simulink model "Model_without_decision_and_sieve"  (R2022a)
settings: Solver=VariableStepAuto  StartTime=0.0  StopTime=1000000  RelTol=1e-3
undefined symbols (not defined in the file): Coefficient_value, Enable_X, Enable_Y, N, s1, s10, s11, s12, s13, s14, s15, s16, s17, s18, s19, s2, s20, s21, s22, s23, s24, s25, s26, s27, s28, s29, s3, s30, s4, s5, s6, s7, s8, s9
libraries: simulink x33
(part 1 of 5)
settings Model: Creator=jhd  LastModifiedBy=AISL
settings SolverCC: AlgebraicLoopSolver=TrustRegion
settings DebuggingCC: UnconnectedInputMsg=warning  UnconnectedOutputMsg=warning  UnconnectedLineMsg=warning  SFMachineParentedDataDiag=warning
settings RTWCC: DLArmComputeVersion=19.05

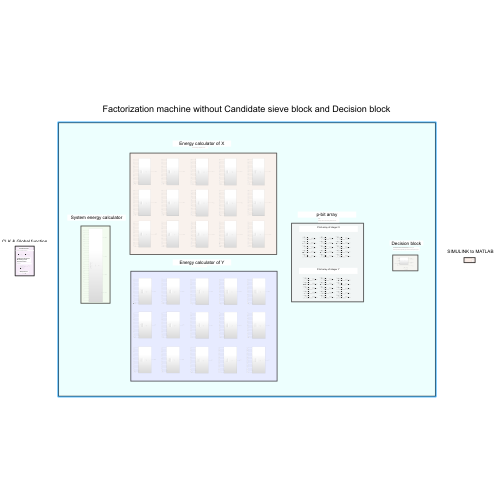
[thumbnail: Simulink's stored preview of the top-level diagram]
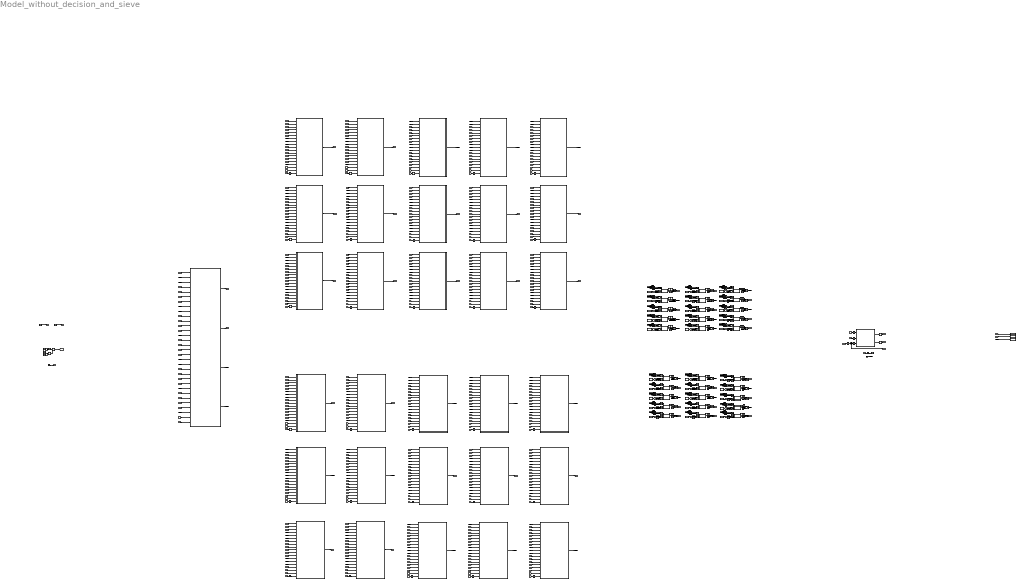
== system Model_without_decision_and_sieve ==
  note: Coefficient value and Bit-shifting of the energy function
  note: UPDATING CLK
  note: P-bit array of integer X
  note: P-bit array of integer Y
  note: CLK & Global function
  note: System energy calculator
  note: Energy calculator of X
  note: Energy calculator of Y
  note: SIMULINK to MATLAB
  note: Decision block
  note: Semiprime N
  note: p-bit array
  note: EN_X, EN_Y, which are signals for updating p-bits.
  note: Calculates the energy for updating the p-bits of X
  note: Calculates the energy for updating the p-bits of Y
  note: When the EN_X(EN_Y) signal rises, the p-bits are updated by the sigmoid function and RNG.
      |
      | Unnecessary number of p-bits for factorizing given N are fixed to zero.
  note: When both X and Y are the factors of semiprime number N, the system energy is 0.
      | Then, the Find signal becomes zero and the simulation stops.
      |
      | In the Enable_switch block, the EN_X and EN_Y signals are fixed to zero when the system energy is 0.
  note: A coefficient value E 0 and bit-shifting operation by the probabilistic annealing method.
  note: Factorization machine without Candidate sieve block and Decision block
  Clock : Clock
  Constant{1..4,6..7,9,11..18,21,29,33,39,57..58,60..61,63..64,66,68..70,72..73,75..76,78..79,81,83,85,87,95,99,101,103..104,106,111,113,117..119,121,123..124,150..151,153..155,195..196} (60 alike) : Constant  Value=0
  Constant10 : Constant  Value=Enable_X(13,1)
  Constant100 : Constant  Value=Enable_X(4,1)
  Constant102 : Constant  Value=Enable_X(3,1)
  Constant105 : Constant  Value=Enable_X(1,1)
  Constant112 : Constant  Value=Enable_X(5,1)
  Constant116 : Constant  Value=Enable_X(2,1)
  Constant120 : Constant  Value=Enable_Y(14,1)
  Constant122 : Constant  Value=Enable_Y(13,1)
  Constant131 : Constant  Value=2
  Constant149 : Constant  Value=Enable_Y(11,1)
  Constant152 : Constant  Value=Enable_Y(12,1)
  Constant194 : Constant  Value=Enable_Y(15,1)
  Constant20 : Constant  Value=Enable_X(11,1)
  Constant22 : Constant  Value=2
  Constant23 : Constant  Value=Coefficient_value
  Constant28 : Constant  Value=Enable_X(15,1)
  Constant32 : Constant  Value=Enable_X(12,1)
  Constant34 : Constant  Value=Enable_X(9,1)
  Constant36 : Constant  Value=Enable_X(8,1)
  Constant5 : Constant  Value=N
  Constant56 : Constant  Value=Enable_Y(4,1)
  Constant59 : Constant  Value=Enable_Y(3,1)
  Constant62 : Constant  Value=Enable_Y(1,1)
  Constant65 : Constant  Value=Enable_Y(5,1)
  Constant67 : Constant  Value=Enable_Y(2,1)
  Constant71 : Constant  Value=Enable_Y(9,1)
  Constant74 : Constant  Value=Enable_Y(8,1)
  Constant77 : Constant  Value=Enable_Y(6,1)
  Constant8 : Constant  Value=Enable_X(14,1)
  Constant80 : Constant  Value=Enable_Y(10,1)
  Constant82 : Constant  Value=Enable_Y(7,1)
  Constant86 : Constant  Value=Enable_X(6,1)
  Constant94 : Constant  Value=Enable_X(10,1)
  Constant98 : Constant  Value=Enable_X(7,1)
  Delay{1..13,17,27..32,34..42,49} (30 alike) : Delay  DelayLength=1
  Enable_Switch : Subsystem
  Logical Operator2 : Logic  Operator=NOT  Inputs=1  AllPortsSameDT=off  OutDataTypeStr=boolean
  Math Function1 : Math  Operator=pow
  Math Function2 : Math  Operator=pow
  Pbit_1 : Subsystem
  Pbit_10 : Subsystem
  Pbit_11 : Subsystem
  Pbit_12 : Subsystem
  Pbit_13 : Subsystem
  Pbit_14 : Subsystem
  Pbit_15 : Subsystem
  Pbit_2 : Subsystem
  Pbit_3 : Subsystem
  Pbit_4 : Subsystem
  Pbit_5 : Subsystem
  Pbit_6 : Subsystem
  Pbit_7 : Subsystem
  Pbit_8 : Subsystem
  Pbit_9 : Subsystem
  Pbit_Y_1 : Subsystem
  Pbit_Y_10 : Subsystem
  Pbit_Y_11 : Subsystem
  Pbit_Y_12 : Subsystem
  Pbit_Y_13 : Subsystem
  Pbit_Y_14 : Subsystem
  Pbit_Y_15 : Subsystem
  Pbit_Y_2 : Subsystem
  Pbit_Y_3 : Subsystem
  Pbit_Y_4 : Subsystem
  Pbit_Y_5 : Subsystem
  Pbit_Y_6 : Subsystem
  Pbit_Y_7 : Subsystem
  Pbit_Y_8 : Subsystem
  Pbit_Y_9 : Subsystem
  Product1 : Product
  Repeating Sequence Stair : simulink/Sources/Repeating Sequence Stair  OutValues=[0 1 2 3].'  tsamp=6  OutMin=[]  OutMax=[]  OutDataTypeStr=double  OutputDataTypeScalingMode=double  OutDataType=fixdt(0,8)  ConRadixGroup=Best Precision: Vector-wise  OutScaling=2^-12
  Repeating Sequence Stair1 : simulink/Sources/Repeating Sequence Stair  OutValues=[1 0 0 0 0 0].'  tsamp=1  OutMin=[]  OutMax=[]  OutDataTypeStr=double  OutputDataTypeScalingMode=double  OutDataType=fixdt(0,8)  ConRadixGroup=Best Precision: Vector-wise  OutScaling=2^-12
  Repeating Sequence Stair2 : simulink/Sources/Repeating Sequence Stair  OutValues=[0 0 0 1 0 0 ].'  tsamp=1  OutMin=[]  OutMax=[]  OutDataTypeStr=double  OutputDataTypeScalingMode=double  OutDataType=fixdt(0,8)  ConRadixGroup=Best Precision: Vector-wise  OutScaling=2^-12
  Stop Simulation : Stop
  Subtract{7..12,17..27,32..39,46..51,56..75,78..84,97..98} (60 alike) : Sum  Inputs=+-
  Switch_{1..3,5..14,28,33,35..36,42,97,102..104,110,112,116..117,122,131,146,174} (30 alike) : Switch  Criteria=u2 ~= 0  OutDataTypeStr=fixdt(0,1,0)  SaturateOnIntegerOverflow=off  InputSameDT=off
  Switch_{4,16,19..20,23,25,29..32,37..41,46,49..50,56,59..60,68..69,77,81,87,89,91,96,98..101,105..109,111,113..115,118..121,123,130,132..133,136..138,140,142,144..145,148,173,175} (60 alike) : Switch  Criteria=u2 ~= 0  SaturateOnIntegerOverflow=off  InputSameDT=off
  Terminator_boundary_DTC1 : DataTypeConversion  OutDataTypeStr=double  RndMeth=Round  SaturateOnIntegerOverflow=off
  Terminator_boundary_DTC{2..21,23..48,59,62,72..74,76..88} (64 alike) : DataTypeConversion  OutDataTypeStr=fixdt(0,1,0)  RndMeth=Round  LockScale=on
  Terminator_boundary_DTC22 : DataTypeConversion  OutDataTypeStr=double  RndMeth=Round  SaturateOnIntegerOverflow=off
  To Workspace1 : ToWorkspace  VariableName=simout1  SampleTime=-1
  To Workspace2 : ToWorkspace  VariableName=simout2  SampleTime=-1
  To Workspace3 : ToWorkspace  VariableName=simout3  SampleTime=-1
  X1 : Subsystem
  X10 : Subsystem
  X11 : Subsystem
  X12 : Subsystem
  X13 : Subsystem
  X14 : Subsystem
  X15 : Subsystem
  X2 : Subsystem
  X3 : Subsystem
  X4 : Subsystem
  X5 : Subsystem
  X6 : Subsystem
  X7 : Subsystem
  X8 : Subsystem
  X9 : Subsystem
  Y : Subsystem
  Y1 : Subsystem
  Y10 : Subsystem
  Y11 : Subsystem
  Y12 : Subsystem
  Y13 : Subsystem
  Y14 : Subsystem
  Y15 : Subsystem
  Y2 : Subsystem
  Y3 : Subsystem
  Y4 : Subsystem
  Y5 : Subsystem
  Y6 : Subsystem
  Y7 : Subsystem
  Y8 : Subsystem
  Y9 : Subsystem
  wires:
  [X] -> To Workspace1/1
  Terminator_boundary_DTC7/1 -> Enable_Switch/1(pre_X)
  [UPDATE_Y] -> Terminator_boundary_DTC2/1
  [UPDATE_X] -> Terminator_boundary_DTC7/1
  Terminator_boundary_DTC1/1 -> [EN_X]
  Terminator_boundary_DTC22/1 -> [EN_Y]
  Terminator_boundary_DTC2/1 -> Enable_Switch/2(pre_Y)
  Enable_Switch/1(EN_X) -> Terminator_boundary_DTC1/1
  Enable_Switch/2(EN_Y) -> Terminator_boundary_DTC22/1
  [Y4] -> Y/19(Y4)
  [Y9] -> Y/24(Y9)
  [Y7] -> Y/22(Y7)
  [Y8] -> Y/23(Y8)
  [Y5] -> Y/20(Y5)
  [Y3] -> Y/18(Y3)
  [Y2] -> Y/17(Y2)
  [Y1] -> Y/16(Y1)
  [Y11] -> Y/26(Y11)
  [Y12] -> Y/27(Y12)
  [Y10] -> Y/25(Y10)
  [Y14] -> Y/29(Y14)
  [Y13] -> Y/28(Y13)
  Terminator_boundary_DTC21/1 -> Enable_Switch/3(energy)
  [Y] -> To Workspace2/1
  [TIME] -> To Workspace3/1
  Repeating Sequence Stair1/1 -> [UPDATE_X]  "UPDATE_X"
  Y/1(E0) -> [E0]
  Repeating Sequence Stair2/1 -> [UPDATE_Y]  "UPDATE_Y"
  [X9] -> X1/9(X9)
  [N] -> X1/17(N)
  Terminator_boundary_DTC59/1 -> X1/19(EN_X)
  [X11] -> X1/11(X11)
  [EN_X] -> Terminator_boundary_DTC59/1
  [X15] -> X1/15(X15)
  [Y] -> X1/16(Y)
  [shifted_coefficient] -> X1/18(shifted_coeff)
  [X7] -> X1/7(X7)
  [X13] -> X1/13(X13)
  X1/1(E_X) -> [E_X1]
  [X12] -> X1/12(X12)
  [X10] -> X1/10(X10)
  [X3] -> X1/3(X3)
  [X5] -> X1/5(X5)
  [X14] -> X1/14(X14)
  [X4] -> X1/4(X4)
  [X6] -> X1/6(X6)
  [X8] -> X1/8(X8)
  [X1] -> X1/1(X1)
  [X2] -> X1/2(X2)
  Y/2(X) -> [X]
  Y/3(Y) -> [Y]
  [Y2] -> Y1/2(Y2)
  [N] -> Y1/17(N)
  [X] -> Y1/16(X)
  [Y1] -> Y1/1(Y1)
  [Y11] -> Y1/11(Y11)
  [EN_Y] -> Terminator_boundary_DTC31/1
  [Y12] -> Y1/12(Y12)
  [Y10] -> Y1/10(Y10)
  [Y3] -> Y1/3(Y3)
  Y1/1(E_Y) -> [E_Y1]
  Terminator_boundary_DTC31/1 -> Y1/19(EN_Y)
  [Y6] -> Y1/6(Y6)
  [shifted_coefficient] -> Y1/18(shifted_coeff)
  [Y4] -> Y1/4(Y4)
  [Y13] -> Y1/13(Y13)
  [Y7] -> Y1/7(Y7)
  [Y5] -> Y1/5(Y5)
  [Y8] -> Y1/8(Y8)
  [X5] -> Y/5(X5)
  [X4] -> Y/4(X4)
  [X6] -> Y/6(X6)
  [X14] -> Y/14(X14)
  [X13] -> Y/13(X13)
  [X7] -> Y/7(X7)
  [X15] -> Y/15(X15)
  [X9] -> Y/9(X9)
  [X2] -> Y/2(X2)
  [X10] -> Y/10(X10)
  [X3] -> Y/3(X3)
  [X12] -> Y/12(X12)
  [X8] -> Y/8(X8)
  Terminator_boundary_DTC87/1 -> [FIND], Terminator_boundary_DTC21/1  "Find"
  Logical Operator2/1 -> Stop Simulation/1
  [FIND] -> Logical Operator2/1
  Clock/1 -> [TIME]
  Y/4(sytem_energy) -> [sytem_energy]  "(XY-N)^2"
  [E0] -> Subtract9/1, Subtract8/2
  [EN_X] -> Switch_16/1
  Constant10/1 -> [EN_X13]
  Subtract20/1 -> Switch_19/3
  Switch_23/1 -> Pbit_15/2(EN)
  [X15] -> Switch_19/2
  [E_X15] -> Subtract20/2, Subtract19/1
  Switch_19/1 -> Pbit_15/1(IN)
  Subtract7/1 -> Switch_56/1
  [E0] -> Subtract20/1, Subtract19/2
  Constant28/1 -> [EN_X15]
  [EN_X15] -> Switch_23/2
  [X14] -> Switch_49/2
  Subtract18/1 -> Switch_49/3
  [E0] -> Subtract17/2, Subtract18/1
  Subtract17/1 -> Switch_49/1
  Subtract19/1 -> Switch_19/1
  [EN_X] -> Switch_46/1
  Constant33/1 -> Switch_46/3
  Switch_4/1 -> Pbit_14/2(EN)
  Switch_46/1 -> Pbit_12/2(EN)
  Constant29/1 -> Switch_23/3
  Constant11/1 -> Switch_16/3
  Switch_56/1 -> Pbit_13/1(IN)
  [EN_X] -> Switch_50/1
  [EN_X12] -> Switch_46/2
  Constant21/1 -> Switch_50/3
  [E_X14] -> Subtract17/1, Subtract18/2
  [X12] -> Switch_20/2
  Switch_20/1 -> Pbit_12/1(IN)
  Subtract10/1 -> Switch_20/1
  [E0] -> Subtract11/1, Subtract10/2
  Constant16/1 -> Switch_4/3
  Switch_50/1 -> Pbit_11/2(EN)
  Subtract12/1 -> Switch_56/3
  [EN_X] -> Switch_23/1
  [EN_X13] -> Switch_16/2
  Switch_16/1 -> Pbit_13/2(EN)
  Subtract8/1 -> Switch_25/1
  [E_X13] -> Subtract7/1, Subtract12/2
  Constant20/1 -> [EN_X11]
  [E_X12] -> Subtract11/2, Subtract10/1
  [X13] -> Switch_56/2
  Switch_49/1 -> Pbit_14/1(IN)
  [E0] -> Subtract7/2, Subtract12/1
  [EN_X14] -> Switch_4/2
  Subtract9/1 -> Switch_25/3
  [EN_X] -> Switch_4/1
  Constant32/1 -> [EN_X12]
  Switch_25/1 -> Pbit_11/1(IN)
  [EN_X11] -> Switch_50/2
  Constant8/1 -> [EN_X14]
  [X11] -> Switch_25/2
  Subtract11/1 -> Switch_20/3
  [E_X11] -> Subtract9/2, Subtract8/1
  [E0] -> Subtract23/1, Subtract22/2
  [EN_X] -> Switch_60/1
  Constant36/1 -> [EN_X8]
  Subtract34/1 -> Switch_68/3
  Switch_77/1 -> Pbit_10/2(EN)
  [X10] -> Switch_68/2
  [E_X10] -> Subtract34/2, Subtract33/1
  Switch_68/1 -> Pbit_10/1(IN)
  Subtract21/1 -> Switch_130/1
  [E0] -> Subtract34/1, Subtract33/2
  Constant94/1 -> [EN_X10]
  [EN_X10] -> Switch_77/2
  [X9] -> Switch_89/2
  Subtract32/1 -> Switch_89/3
  [E0] -> Subtract27/2, Subtract32/1
  Subtract27/1 -> Switch_89/1
  Subtract33/1 -> Switch_68/1
  [EN_X] -> Switch_87/1
  Constant99/1 -> Switch_87/3
  Switch_59/1 -> Pbit_9/2(EN)
  Switch_87/1 -> Pbit_7/2(EN)
  Constant95/1 -> Switch_77/3
  Constant39/1 -> Switch_60/3
  Switch_130/1 -> Pbit_8/1(IN)
  [EN_X] -> Switch_91/1
  [EN_X7] -> Switch_87/2
  Constant87/1 -> Switch_91/3
  [E_X9] -> Subtract27/1, Subtract32/2
  [X7] -> Switch_69/2
  Switch_69/1 -> Pbit_7/1(IN)
  Subtract24/1 -> Switch_69/1
  [E0] -> Subtract25/1, Subtract24/2
  Constant85/1 -> Switch_59/3
  Switch_91/1 -> Pbit_6/2(EN)
  Subtract26/1 -> Switch_130/3
  [EN_X] -> Switch_77/1
  [EN_X8] -> Switch_60/2
  Switch_60/1 -> Pbit_8/2(EN)
  Subtract22/1 -> Switch_81/1
  [E_X8] -> Subtract21/1, Subtract26/2
  Constant86/1 -> [EN_X6]
  [E_X7] -> Subtract25/2, Subtract24/1
  [X8] -> Switch_130/2
  Switch_89/1 -> Pbit_9/1(IN)
  [E0] -> Subtract21/2, Subtract26/1
  [EN_X9] -> Switch_59/2
  Subtract23/1 -> Switch_81/3
  [EN_X] -> Switch_59/1
  Constant98/1 -> [EN_X7]
  Switch_81/1 -> Pbit_6/1(IN)
  [EN_X6] -> Switch_91/2
  Constant34/1 -> [EN_X9]
  [X6] -> Switch_81/2
  Subtract25/1 -> Switch_69/3
  [E_X6] -> Subtract23/2, Subtract22/1
  Pbit_2/1(OUT) -> Delay17/1
  [E0] -> Subtract37/1, Subtract36/2
  [EN_X] -> Switch_133/1
  Constant102/1 -> [EN_X3]
  [EN_X1] -> Switch_131/2
  Constant111/1 -> Switch_131/3
  Delay42/1 -> Terminator_boundary_DTC62/1
  Switch_131/1 -> [X1]
  Subtract84/1 -> Switch_136/3
  Switch_138/1 -> Pbit_5/2(EN)
  [X5] -> Switch_136/2
  [E_X5] -> Subtract84/2, Subtract59/1
  Switch_136/1 -> Pbit_5/1(IN)
  Subtract35/1 -> Switch_148/1
  [E0] -> Subtract84/1, Subtract59/2
  Constant112/1 -> [EN_X5]
  [EN_X5] -> Switch_138/2
  [X4] -> Switch_144/2
  Terminator_boundary_DTC62/1 -> Switch_131/1
  Subtract58/1 -> Switch_144/3
  [E0] -> Subtract57/2, Subtract58/1
  Subtract57/1 -> Switch_144/1
  Subtract59/1 -> Switch_136/1
  [EN_X] -> Switch_142/1
  Constant117/1 -> Switch_142/3
  Switch_132/1 -> Pbit_4/2(EN)
  Switch_142/1 -> Pbit_2/2(EN)
  Constant113/1 -> Switch_138/3
  Constant103/1 -> Switch_133/3
  Pbit_1/1(OUT) -> Delay42/1
  [EN_X2] -> Switch_142/2
  Constant106/1 -> Switch_145/3
  [E_X4] -> Subtract57/1, Subtract58/2
  Constant101/1 -> Switch_146/3
  [EN_X2] -> Switch_146/2
  [X2] -> Switch_137/2
  Switch_137/1 -> Pbit_2/1(IN)
  Subtract38/1 -> Switch_137/1
  Delay17/1 -> Terminator_boundary_DTC76/1
  [E0] -> Subtract39/1, Subtract38/2
  [EN_X] -> Switch_132/1
  Constant116/1 -> [EN_X2]
  Switch_146/1 -> [X2]
  Constant104/1 -> Switch_132/3
  Terminator_boundary_DTC76/1 -> Switch_146/1
  Constant100/1 -> [EN_X4]
  Switch_145/1 -> Pbit_1/2(EN)
  [EN_X1] -> Switch_145/2
  Subtract56/1 -> Switch_148/3
  [EN_X] -> Switch_138/1
  [E_X3] -> Subtract35/1, Subtract56/2
  [EN_X3] -> Switch_133/2
  Switch_133/1 -> Pbit_3/2(EN)
  Subtract36/1 -> Switch_140/1
  Constant105/1 -> [EN_X1]
  [E_X2] -> Subtract39/2, Subtract38/1
  [X3] -> Switch_148/2
  Switch_144/1 -> Pbit_4/1(IN)
  [E0] -> Subtract35/2, Subtract56/1
  [EN_X4] -> Switch_132/2
  Switch_148/1 -> Pbit_3/1(IN)
  Subtract37/1 -> Switch_140/3
  [EN_X] -> Switch_145/1
  Switch_140/1 -> Pbit_1/1(IN)
  [E_X1] -> Subtract37/2, Subtract36/1
  [X1] -> Switch_140/2
  Subtract39/1 -> Switch_137/3
  Pbit_Y_2/1(OUT) -> Delay28/1
  [E0] -> Subtract48/1, Subtract47/2
  [EN_Y] -> Switch_30/1
  Constant59/1 -> [EN_Y3]
  [EN_Y1] -> Switch_28/2
  Constant64/1 -> Switch_28/3
  Delay31/1 -> Terminator_boundary_DTC72/1
  Switch_28/1 -> [Y1]
  Subtract63/1 -> Switch_31/3
  Switch_37/1 -> Pbit_Y_5/2(EN)
  [Y5] -> Switch_31/2
  [E_Y5] -> Subtract63/2, Subtract62/1
  Switch_31/1 -> Pbit_Y_5/1(IN)
  Subtract46/1 -> Switch_96/1
  [E0] -> Subtract63/1, Subtract62/2
  Constant65/1 -> [EN_Y5]
  [EN_Y5] -> Switch_37/2
  [Y4] -> Switch_40/2
  Terminator_boundary_DTC72/1 -> Switch_28/1
  Subtract61/1 -> Switch_40/3
  [E0] -> Subtract60/2, Subtract61/1
  Subtract60/1 -> Switch_40/1
  Subtract62/1 -> Switch_31/1
  [EN_Y] -> Switch_39/1
  Constant68/1 -> Switch_39/3
  Switch_29/1 -> Pbit_Y_4/2(EN)
  Switch_39/1 -> Pbit_Y_2/2(EN)
  Constant66/1 -> Switch_37/3
  Terminator_boundary_DTC74/1 -> Switch_35/1
  Switch_35/1 -> [Y4]
  [EN_Y4] -> Switch_35/2
  Pbit_Y_1/1(OUT) -> Delay31/1
  [EN_Y2] -> Switch_39/2
  Pbit_Y_5/1(OUT) -> Delay30/1
  Constant63/1 -> Switch_41/3
  Constant58/1 -> Switch_42/3
  [EN_Y2] -> Switch_42/2
  Switch_42/1 -> [Y2]
  Constant57/1 -> Switch_36/3
  [EN_Y5] -> Switch_36/2
  [E_Y4] -> Subtract60/1, Subtract61/2
  Switch_36/1 -> [Y5]
  Terminator_boundary_DTC77/1 -> Switch_36/1
  Pbit_Y_3/1(OUT) -> Delay27/1
  [Y2] -> Switch_32/2
  Constant70/1 -> Switch_35/3
  Switch_32/1 -> Pbit_Y_2/1(IN)
  Subtract49/1 -> Switch_32/1
  Pbit_Y_4/1(OUT) -> Delay29/1
  Delay28/1 -> Terminator_boundary_DTC78/1
  [E0] -> Subtract50/1, Subtract49/2
  Switch_40/1 -> Pbit_Y_4/1(IN)
  [EN_Y] -> Switch_29/1
  Constant67/1 -> [EN_Y2]
  Constant61/1 -> Switch_29/3
  Terminator_boundary_DTC78/1 -> Switch_42/1
  Constant56/1 -> [EN_Y4]
  Switch_41/1 -> Pbit_Y_1/2(EN)
  Delay27/1 -> Terminator_boundary_DTC73/1
  Constant69/1 -> Switch_33/3
  [EN_Y1] -> Switch_41/2
  Subtract51/1 -> Switch_96/3
  Delay29/1 -> Terminator_boundary_DTC74/1
  [EN_Y] -> Switch_37/1
  [E_Y3] -> Subtract46/1, Subtract51/2
  Delay30/1 -> Terminator_boundary_DTC77/1
  [EN_Y3] -> Switch_30/2
  Switch_30/1 -> Pbit_Y_3/2(EN)
  Subtract47/1 -> Switch_38/1
  Constant62/1 -> [EN_Y1]
  [EN_Y3] -> Switch_33/2
  [E_Y2] -> Subtract50/2, Subtract49/1
  Switch_33/1 -> [Y3]
  [Y3] -> Switch_96/2
  [E0] -> Subtract46/2, Subtract51/1
  [EN_Y4] -> Switch_29/2
  Switch_96/1 -> Pbit_Y_3/1(IN)
  Subtract48/1 -> Switch_38/3
  [EN_Y] -> Switch_41/1
  Switch_38/1 -> Pbit_Y_1/1(IN)
  [E_Y1] -> Subtract48/2, Subtract47/1
  Constant60/1 -> Switch_30/3
  [Y1] -> Switch_38/2
  Terminator_boundary_DTC73/1 -> Switch_33/1
  Subtract50/1 -> Switch_32/3
  Pbit_Y_7/1(OUT) -> Delay34/1
  [E0] -> Subtract66/1, Subtract65/2
  [EN_Y] -> Switch_99/1
  Constant74/1 -> [EN_Y8]
  [EN_Y6] -> Switch_97/2
  Constant79/1 -> Switch_97/3
  Delay37/1 -> Terminator_boundary_DTC79/1
  Switch_97/1 -> [Y6]
  Subtract73/1 -> Switch_100/3
  Switch_105/1 -> Pbit_Y_10/2(EN)
  [Y10] -> Switch_100/2
  [E_Y10] -> Subtract73/2, Subtract72/1
  Switch_100/1 -> Pbit_Y_10/1(IN)
  Subtract64/1 -> Switch_111/1
  [E0] -> Subtract73/1, Subtract72/2
  Constant80/1 -> [EN_Y10]
  [EN_Y10] -> Switch_105/2
  [Y9] -> Switch_108/2
  Terminator_boundary_DTC79/1 -> Switch_97/1
  Subtract71/1 -> Switch_108/3
  [E0] -> Subtract70/2, Subtract71/1
  Subtract70/1 -> Switch_108/1
  Subtract72/1 -> Switch_100/1
  [EN_Y] -> Switch_107/1
  Constant83/1 -> Switch_107/3
  Switch_98/1 -> Pbit_Y_9/2(EN)
  Switch_107/1 -> Pbit_Y_7/2(EN)
  Constant81/1 -> Switch_105/3
  Terminator_boundary_DTC81/1 -> Switch_103/1
  Switch_103/1 -> [Y9]
  [EN_Y9] -> Switch_103/2
  Pbit_Y_6/1(OUT) -> Delay37/1
  [EN_Y7] -> Switch_107/2
  Pbit_Y_10/1(OUT) -> Delay36/1
  Constant78/1 -> Switch_109/3
  Constant73/1 -> Switch_110/3
  [EN_Y7] -> Switch_110/2
  Switch_110/1 -> [Y7]
  Constant72/1 -> Switch_104/3
  [EN_Y10] -> Switch_104/2
  [E_Y9] -> Subtract70/1, Subtract71/2
  Switch_104/1 -> [Y10]
  Terminator_boundary_DTC82/1 -> Switch_104/1
  Pbit_Y_8/1(OUT) -> Delay32/1
  [Y7] -> Switch_101/2
  Constant119/1 -> Switch_103/3
  Switch_101/1 -> Pbit_Y_7/1(IN)
  Subtract67/1 -> Switch_101/1
  Pbit_Y_9/1(OUT) -> Delay35/1
  Delay34/1 -> Terminator_boundary_DTC83/1
  [E0] -> Subtract68/1, Subtract67/2
  Switch_108/1 -> Pbit_Y_9/1(IN)
  [EN_Y] -> Switch_98/1
  Constant82/1 -> [EN_Y7]
  Constant76/1 -> Switch_98/3
  Terminator_boundary_DTC83/1 -> Switch_110/1
  Constant71/1 -> [EN_Y9]
  Switch_109/1 -> Pbit_Y_6/2(EN)
  Delay32/1 -> Terminator_boundary_DTC80/1
  Constant118/1 -> Switch_102/3
  [EN_Y6] -> Switch_109/2
  Subtract69/1 -> Switch_111/3
  Delay35/1 -> Terminator_boundary_DTC81/1
  [EN_Y] -> Switch_105/1
  [E_Y8] -> Subtract64/1, Subtract69/2
  Delay36/1 -> Terminator_boundary_DTC82/1
  [EN_Y8] -> Switch_99/2
  Switch_99/1 -> Pbit_Y_8/2(EN)
  Subtract65/1 -> Switch_106/1
  Constant77/1 -> [EN_Y6]
  [EN_Y8] -> Switch_102/2
  [E_Y7] -> Subtract68/2, Subtract67/1
  Switch_102/1 -> [Y8]
  [Y8] -> Switch_111/2
  [E0] -> Subtract64/2, Subtract69/1
  [EN_Y9] -> Switch_98/2
  Switch_111/1 -> Pbit_Y_8/1(IN)
  Subtract66/1 -> Switch_106/3
  [EN_Y] -> Switch_109/1
  Switch_106/1 -> Pbit_Y_6/1(IN)
  [E_Y6] -> Subtract66/2, Subtract65/1
  Constant75/1 -> Switch_99/3
  [Y6] -> Switch_106/2
  Terminator_boundary_DTC80/1 -> Switch_102/1
  Subtract68/1 -> Switch_101/3
  Pbit_Y_12/1(OUT) -> Delay39/1
  [E0] -> Subtract78/1, Subtract75/2
  Subtract74/1 -> Switch_123/1
  [EN_Y] -> Switch_114/1
  Constant122/1 -> [EN_Y13]
  [EN_Y11] -> Switch_112/2
  Constant151/1 -> Switch_112/3
  Delay41/1 -> Terminator_boundary_DTC84/1
  Switch_112/1 -> [Y11]
  [Y14] -> Switch_120/2
  Terminator_boundary_DTC84/1 -> Switch_112/1
  Subtract83/1 -> Switch_120/3
  [E0] -> Subtract82/2, Subtract83/1
  Subtract82/1 -> Switch_120/1
  [EN_Y] -> Switch_119/1
  Constant153/1 -> Switch_119/3
  Switch_119/1 -> Pbit_Y_12/2(EN)
  Switch_117/1 -> [Y14]
  [EN_Y14] -> Switch_117/2
  Pbit_Y_11/1(OUT) -> Delay41/1
  [EN_Y12] -> Switch_119/2
  Constant150/1 -> Switch_121/3
  [E_Y14] -> Subtract82/1, Subtract83/2
  Constant121/1 -> Switch_122/3
  [EN_Y12] -> Switch_122/2
  Switch_122/1 -> [Y12]
  Pbit_Y_13/1(OUT) -> Delay38/1
  [Y12] -> Switch_115/2
  Switch_115/1 -> Pbit_Y_12/1(IN)
  Constant155/1 -> Switch_117/3
  Subtract79/1 -> Switch_115/1
  Pbit_Y_14/1(OUT) -> Delay40/1
  Terminator_boundary_DTC86/1 -> Switch_117/1
  Delay39/1 -> Terminator_boundary_DTC88/1
  [E0] -> Subtract80/1, Subtract79/2
  Switch_120/1 -> Pbit_Y_14/1(IN)
  [EN_Y] -> Switch_113/1
  Constant152/1 -> [EN_Y12]
  Constant124/1 -> Switch_113/3
  Terminator_boundary_DTC88/1 -> Switch_122/1
  Constant120/1 -> [EN_Y14]
  Switch_121/1 -> Pbit_Y_11/2(EN)
  Delay38/1 -> Terminator_boundary_DTC85/1
  Constant154/1 -> Switch_116/3
  [EN_Y11] -> Switch_121/2
  Subtract81/1 -> Switch_123/3
  Delay40/1 -> Terminator_boundary_DTC86/1
  [E_Y13] -> Subtract74/1, Subtract81/2
  Switch_113/1 -> Pbit_Y_14/2(EN)
  [EN_Y13] -> Switch_114/2
  Switch_114/1 -> Pbit_Y_13/2(EN)
  Subtract75/1 -> Switch_118/1
  Constant149/1 -> [EN_Y11]
  [EN_Y13] -> Switch_116/2
  [E_Y12] -> Subtract80/2, Subtract79/1
  Switch_116/1 -> [Y13]
  [Y13] -> Switch_123/2
  [E0] -> Subtract74/2, Subtract81/1
  [EN_Y14] -> Switch_113/2
  Switch_123/1 -> Pbit_Y_13/1(IN)
  Subtract78/1 -> Switch_118/3
  [EN_Y] -> Switch_121/1
  Switch_118/1 -> Pbit_Y_11/1(IN)
  [E_Y11] -> Subtract78/2, Subtract75/1
  Constant123/1 -> Switch_114/3
  [Y11] -> Switch_118/2
  Terminator_boundary_DTC85/1 -> Switch_116/1
  Subtract80/1 -> Switch_115/3
  [Y15] -> Y/30(Y15)
  [shifted_coefficient] -> Y/32(shifted_coeff)
  [N] -> Y/31(N)
  [Y6] -> Y/21(Y6)
  [X11] -> Y/11(X11)
  [X1] -> Y/1(X1)
  [Y9] -> Y1/9(Y9)
  [Y14] -> Y1/14(Y14)
  [Y15] -> Y1/15(Y15)
  [EN_Y15] -> Switch_173/2
  Subtract97/1 -> Switch_175/1
  [EN_Y15] -> Switch_174/2
  [EN_Y] -> Switch_173/1
  Constant195/1 -> Switch_173/3
  Constant196/1 -> Switch_174/3
  Switch_175/1 -> Pbit_Y_15/1(IN)
  Pbit_Y_15/1(OUT) -> Delay49/1
  [E_Y15] -> Subtract97/1, Subtract98/2
  [E0] -> Subtract97/2, Subtract98/1
  Delay49/1 -> Terminator_boundary_DTC10/1
  Subtract98/1 -> Switch_175/3
  Constant194/1 -> [EN_Y15]
  Switch_174/1 -> [Y15]
  Switch_173/1 -> Pbit_Y_15/2(EN)
  Terminator_boundary_DTC10/1 -> Switch_174/1
  [Y15] -> Switch_175/2
  [X2] -> X2/2(X2)
  [X1] -> X2/1(X1)
  [X8] -> X2/8(X8)
  [X6] -> X2/6(X6)
  [X4] -> X2/4(X4)
  [X14] -> X2/14(X14)
  [X5] -> X2/5(X5)
  [X3] -> X2/3(X3)
  [X10] -> X2/10(X10)
  [X12] -> X2/12(X12)
  X2/1(E_X) -> [E_X2]
  [X13] -> X2/13(X13)
  [X7] -> X2/7(X7)
  [shifted_coefficient] -> X2/18(shifted_coeff)
  [Y] -> X2/16(Y)
  [X15] -> X2/15(X15)
  [EN_X] -> Terminator_boundary_DTC19/1
  [X11] -> X2/11(X11)
  Terminator_boundary_DTC19/1 -> X2/19(EN_X)
  [N] -> X2/17(N)
  [X9] -> X2/9(X9)
  [X9] -> X4/9(X9)
  [N] -> X4/17(N)
  Terminator_boundary_DTC20/1 -> X4/19(EN_X)
  [X11] -> X4/11(X11)
  [EN_X] -> Terminator_boundary_DTC20/1
  [X15] -> X4/15(X15)
  [Y] -> X4/16(Y)
  [shifted_coefficient] -> X4/18(shifted_coeff)
  [X7] -> X4/7(X7)
  [X13] -> X4/13(X13)
  X4/1(E_X) -> [E_X4]
  [X12] -> X4/12(X12)
  [X10] -> X4/10(X10)
  [X3] -> X4/3(X3)
  [X5] -> X4/5(X5)
  [X14] -> X4/14(X14)
  [X4] -> X4/4(X4)
  [X6] -> X4/6(X6)
  [X8] -> X4/8(X8)
  [X1] -> X4/1(X1)
  [X2] -> X4/2(X2)
  [X2] -> X3/2(X2)
  [X1] -> X3/1(X1)
  [X8] -> X3/8(X8)
  [X6] -> X3/6(X6)
  [X4] -> X3/4(X4)
  [X14] -> X3/14(X14)
  [X5] -> X3/5(X5)
  [X3] -> X3/3(X3)
  [X10] -> X3/10(X10)
  [X12] -> X3/12(X12)
  X3/1(E_X) -> [E_X3]
  [X13] -> X3/13(X13)
  [X7] -> X3/7(X7)
  [shifted_coefficient] -> X3/18(shifted_coeff)
  [Y] -> X3/16(Y)
  [X15] -> X3/15(X15)
  [EN_X] -> Terminator_boundary_DTC23/1
  [X11] -> X3/11(X11)
  Terminator_boundary_DTC23/1 -> X3/19(EN_X)
  [N] -> X3/17(N)
  [X9] -> X3/9(X9)
  [X2] -> X5/2(X2)
  [X1] -> X5/1(X1)
  [X8] -> X5/8(X8)
  [X6] -> X5/6(X6)
  [X4] -> X5/4(X4)
  [X14] -> X5/14(X14)
  [X5] -> X5/5(X5)
  [X3] -> X5/3(X3)
  [X10] -> X5/10(X10)
  [X12] -> X5/12(X12)
  X5/1(E_X) -> [E_X5]
  [X13] -> X5/13(X13)
  [X7] -> X5/7(X7)
  [shifted_coefficient] -> X5/18(shifted_coeff)
  [Y] -> X5/16(Y)
  [X15] -> X5/15(X15)
  [EN_X] -> Terminator_boundary_DTC24/1
  [X11] -> X5/11(X11)
  Terminator_boundary_DTC24/1 -> X5/19(EN_X)
  [N] -> X5/17(N)
  [X9] -> X5/9(X9)
  [X9] -> X10/9(X9)
  [N] -> X10/17(N)
  Terminator_boundary_DTC28/1 -> X10/19(EN_X)
  [X11] -> X10/11(X11)
  [EN_X] -> Terminator_boundary_DTC28/1
  [X15] -> X10/15(X15)
  [Y] -> X10/16(Y)
  [shifted_coefficient] -> X10/18(shifted_coeff)
  [X7] -> X10/7(X7)
  [X13] -> X10/13(X13)
  X10/1(E_X) -> [E_X10]
  [X12] -> X10/12(X12)
  [X10] -> X10/10(X10)
  [X3] -> X10/3(X3)
  [X5] -> X10/5(X5)
  [X14] -> X10/14(X14)
  [X4] -> X10/4(X4)
  [X6] -> X10/6(X6)
  [X8] -> X10/8(X8)
  [X1] -> X10/1(X1)
  [X2] -> X10/2(X2)
  [X9] -> X8/9(X9)
  [N] -> X8/17(N)
  Terminator_boundary_DTC27/1 -> X8/19(EN_X)
  [X11] -> X8/11(X11)
  [EN_X] -> Terminator_boundary_DTC27/1
  [X15] -> X8/15(X15)
  [Y] -> X8/16(Y)
  [shifted_coefficient] -> X8/18(shifted_coeff)
  [X7] -> X8/7(X7)
  [X13] -> X8/13(X13)
  X8/1(E_X) -> [E_X8]
  [X12] -> X8/12(X12)
  [X10] -> X8/10(X10)
  [X3] -> X8/3(X3)
  [X5] -> X8/5(X5)
  [X14] -> X8/14(X14)
  [X4] -> X8/4(X4)
  [X6] -> X8/6(X6)
  [X8] -> X8/8(X8)
  [X1] -> X8/1(X1)
  [X2] -> X8/2(X2)
  [X2] -> X9/2(X2)
  [X1] -> X9/1(X1)
  [X8] -> X9/8(X8)
  [X6] -> X9/6(X6)
  [X4] -> X9/4(X4)
  [X14] -> X9/14(X14)
  [X5] -> X9/5(X5)
  [X3] -> X9/3(X3)
  [X10] -> X9/10(X10)
  [X12] -> X9/12(X12)
  X9/1(E_X) -> [E_X9]
  [X13] -> X9/13(X13)
  [X7] -> X9/7(X7)
  [shifted_coefficient] -> X9/18(shifted_coeff)
  [Y] -> X9/16(Y)
  [X15] -> X9/15(X15)
  [EN_X] -> Terminator_boundary_DTC26/1
  [X11] -> X9/11(X11)
  Terminator_boundary_DTC26/1 -> X9/19(EN_X)
  [N] -> X9/17(N)
  [X9] -> X9/9(X9)
  [X9] -> X7/9(X9)
  [N] -> X7/17(N)
  Terminator_boundary_DTC25/1 -> X7/19(EN_X)
  [X11] -> X7/11(X11)
  [EN_X] -> Terminator_boundary_DTC25/1
  [X15] -> X7/15(X15)
  [Y] -> X7/16(Y)
  [shifted_coefficient] -> X7/18(shifted_coeff)
  [X7] -> X7/7(X7)
  [X13] -> X7/13(X13)
  X7/1(E_X) -> [E_X7]
  [X12] -> X7/12(X12)
  [X10] -> X7/10(X10)
  [X3] -> X7/3(X3)
  [X5] -> X7/5(X5)
  [X14] -> X7/14(X14)
  [X4] -> X7/4(X4)
  [X6] -> X7/6(X6)
  [X8] -> X7/8(X8)
  [X1] -> X7/1(X1)
  [X2] -> X7/2(X2)
  [X2] -> X6/2(X2)
  [X1] -> X6/1(X1)
  [X8] -> X6/8(X8)
  [X6] -> X6/6(X6)
  [X4] -> X6/4(X4)
  [X14] -> X6/14(X14)
  [X5] -> X6/5(X5)
  [X3] -> X6/3(X3)
  [X10] -> X6/10(X10)
  [X12] -> X6/12(X12)
  X6/1(E_X) -> [E_X6]
  [X13] -> X6/13(X13)
  [X7] -> X6/7(X7)
  [shifted_coefficient] -> X6/18(shifted_coeff)
  [Y] -> X6/16(Y)
  [X15] -> X6/15(X15)
  [EN_X] -> Terminator_boundary_DTC29/1
  [X11] -> X6/11(X11)
  Terminator_boundary_DTC29/1 -> X6/19(EN_X)
  [N] -> X6/17(N)
  [X9] -> X6/9(X9)
  [X9] -> X15/9(X9)
  [N] -> X15/17(N)
  Terminator_boundary_DTC34/1 -> X15/19(EN_X)
  [X11] -> X15/11(X11)
  [EN_X] -> Terminator_boundary_DTC34/1
  [X15] -> X15/15(X15)
  [Y] -> X15/16(Y)
  [shifted_coefficient] -> X15/18(shifted_coeff)
  [X7] -> X15/7(X7)
  [X13] -> X15/13(X13)
  X15/1(E_X) -> [E_X15]
  [X12] -> X15/12(X12)
  [X10] -> X15/10(X10)
  [X3] -> X15/3(X3)
  [X5] -> X15/5(X5)
  [X14] -> X15/14(X14)
  [X4] -> X15/4(X4)
  [X6] -> X15/6(X6)
  [X8] -> X15/8(X8)
  [X1] -> X15/1(X1)
  [X2] -> X15/2(X2)
  [X9] -> X13/9(X9)
  [N] -> X13/17(N)
  Terminator_boundary_DTC33/1 -> X13/19(EN_X)
  [X11] -> X13/11(X11)
  [EN_X] -> Terminator_boundary_DTC33/1
  [X15] -> X13/15(X15)
  [Y] -> X13/16(Y)
  [shifted_coefficient] -> X13/18(shifted_coeff)
  [X7] -> X13/7(X7)
  [X13] -> X13/13(X13)
  X13/1(E_X) -> [E_X13]
  [X12] -> X13/12(X12)
  [X10] -> X13/10(X10)
  [X3] -> X13/3(X3)
  [X5] -> X13/5(X5)
  [X14] -> X13/14(X14)
  [X4] -> X13/4(X4)
  [X6] -> X13/6(X6)
  [X8] -> X13/8(X8)
  [X1] -> X13/1(X1)
  [X2] -> X13/2(X2)
  [X2] -> X14/2(X2)
  [X1] -> X14/1(X1)
  [X8] -> X14/8(X8)
  [X6] -> X14/6(X6)
  [X4] -> X14/4(X4)
  [X14] -> X14/14(X14)
  [X5] -> X14/5(X5)
  [X3] -> X14/3(X3)
  [X10] -> X14/10(X10)
  [X12] -> X14/12(X12)
  X14/1(E_X) -> [E_X14]
  [X13] -> X14/13(X13)
  [X7] -> X14/7(X7)
  [shifted_coefficient] -> X14/18(shifted_coeff)
  [Y] -> X14/16(Y)
  [X15] -> X14/15(X15)
  [EN_X] -> Terminator_boundary_DTC32/1
  [X11] -> X14/11(X11)
  Terminator_boundary_DTC32/1 -> X14/19(EN_X)
  [N] -> X14/17(N)
  [X9] -> X14/9(X9)
  [X9] -> X12/9(X9)
  [N] -> X12/17(N)
  Terminator_boundary_DTC30/1 -> X12/19(EN_X)
  [X11] -> X12/11(X11)
  [EN_X] -> Terminator_boundary_DTC30/1
  [X15] -> X12/15(X15)
  [Y] -> X12/16(Y)
  [shifted_coefficient] -> X12/18(shifted_coeff)
  [X7] -> X12/7(X7)
  [X13] -> X12/13(X13)
  X12/1(E_X) -> [E_X12]
  [X12] -> X12/12(X12)
  [X10] -> X12/10(X10)
  [X3] -> X12/3(X3)
  [X5] -> X12/5(X5)
  [X14] -> X12/14(X14)
  [X4] -> X12/4(X4)
  [X6] -> X12/6(X6)
  [X8] -> X12/8(X8)
  [X1] -> X12/1(X1)
  [X2] -> X12/2(X2)
  [X2] -> X11/2(X2)
  [X1] -> X11/1(X1)
  [X8] -> X11/8(X8)
  [X6] -> X11/6(X6)
  [X4] -> X11/4(X4)
  [X14] -> X11/14(X14)
  [X5] -> X11/5(X5)
  [X3] -> X11/3(X3)
  [X10] -> X11/10(X10)
  [X12] -> X11/12(X12)
  X11/1(E_X) -> [E_X11]
  [X13] -> X11/13(X13)
  [X7] -> X11/7(X7)
  [shifted_coefficient] -> X11/18(shifted_coeff)
  [Y] -> X11/16(Y)
  [X15] -> X11/15(X15)
  [EN_X] -> Terminator_boundary_DTC40/1
  [X11] -> X11/11(X11)
  Terminator_boundary_DTC40/1 -> X11/19(EN_X)
  [N] -> X11/17(N)
  [X9] -> X11/9(X9)
  Y2/1(E_Y) -> [E_Y2]
  Y3/1(E_Y) -> [E_Y3]
  Y4/1(E_Y) -> [E_Y4]
  Y5/1(E_Y) -> [E_Y5]
  Y10/1(E_Y) -> [E_Y10]
  Y9/1(E_Y) -> [E_Y9]
  Y8/1(E_Y) -> [E_Y8]
  Y7/1(E_Y) -> [E_Y7]
  Y6/1(E_Y) -> [E_Y6]
  Y15/1(E_Y) -> [E_Y15]
  Y14/1(E_Y) -> [E_Y14]
  Y13/1(E_Y) -> [E_Y13]
  Y12/1(E_Y) -> [E_Y12]
  Y11/1(E_Y) -> [E_Y11]
  [sytem_energy] -> Terminator_boundary_DTC87/1
  Constant5/1 -> [N]
  [EN_Y] -> Terminator_boundary_DTC3/1
  [N] -> Y2/17(N)
  [shifted_coefficient] -> Y2/18(shifted_coeff)
  [Y15] -> Y2/15(Y15)
  [Y6] -> Y2/6(Y6)
  [Y13] -> Y2/13(Y13)
  [Y5] -> Y2/5(Y5)
  [Y14] -> Y2/14(Y14)
  [Y4] -> Y2/4(Y4)
  [Y7] -> Y2/7(Y7)
  [Y8] -> Y2/8(Y8)
  [Y12] -> Y2/12(Y12)
  [Y2] -> Y2/2(Y2)
  [Y11] -> Y2/11(Y11)
  [Y9] -> Y2/9(Y9)
  [Y3] -> Y2/3(Y3)
  [X] -> Y2/16(X)
  [Y10] -> Y2/10(Y10)
  [Y1] -> Y2/1(Y1)
  Terminator_boundary_DTC3/1 -> Y2/19(EN_Y)
  [EN_Y] -> Terminator_boundary_DTC4/1
  [N] -> Y3/17(N)
  [shifted_coefficient] -> Y3/18(shifted_coeff)
  [Y15] -> Y3/15(Y15)
  [Y6] -> Y3/6(Y6)
  [Y13] -> Y3/13(Y13)
  [Y5] -> Y3/5(Y5)
  [Y14] -> Y3/14(Y14)
  [Y4] -> Y3/4(Y4)
  [Y7] -> Y3/7(Y7)
  [Y8] -> Y3/8(Y8)
  [Y12] -> Y3/12(Y12)
  [Y2] -> Y3/2(Y2)
  [Y11] -> Y3/11(Y11)
  [Y9] -> Y3/9(Y9)
  [Y3] -> Y3/3(Y3)
  [X] -> Y3/16(X)
  [Y10] -> Y3/10(Y10)
  [Y1] -> Y3/1(Y1)
  Terminator_boundary_DTC4/1 -> Y3/19(EN_Y)
  [EN_Y] -> Terminator_boundary_DTC5/1
  [N] -> Y4/17(N)
  [shifted_coefficient] -> Y4/18(shifted_coeff)
  [Y15] -> Y4/15(Y15)
  [Y6] -> Y4/6(Y6)
  [Y13] -> Y4/13(Y13)
  [Y5] -> Y4/5(Y5)
  [Y14] -> Y4/14(Y14)
  [Y4] -> Y4/4(Y4)
  [Y7] -> Y4/7(Y7)
  [Y8] -> Y4/8(Y8)
  [Y12] -> Y4/12(Y12)
  [Y2] -> Y4/2(Y2)
  [Y11] -> Y4/11(Y11)
  [Y9] -> Y4/9(Y9)
  [Y3] -> Y4/3(Y3)
  [X] -> Y4/16(X)
  [Y10] -> Y4/10(Y10)
  [Y1] -> Y4/1(Y1)
  Terminator_boundary_DTC5/1 -> Y4/19(EN_Y)
  [EN_Y] -> Terminator_boundary_DTC6/1
  [N] -> Y5/17(N)
  [shifted_coefficient] -> Y5/18(shifted_coeff)
  [Y15] -> Y5/15(Y15)
  [Y6] -> Y5/6(Y6)
  [Y13] -> Y5/13(Y13)
  [Y5] -> Y5/5(Y5)
  [Y14] -> Y5/14(Y14)
  [Y4] -> Y5/4(Y4)
  [Y7] -> Y5/7(Y7)
  [Y8] -> Y5/8(Y8)
  [Y12] -> Y5/12(Y12)
  [Y2] -> Y5/2(Y2)
  [Y11] -> Y5/11(Y11)
  [Y9] -> Y5/9(Y9)
  [Y3] -> Y5/3(Y3)
  [X] -> Y5/16(X)
  [Y10] -> Y5/10(Y10)
  [Y1] -> Y5/1(Y1)
  Terminator_boundary_DTC6/1 -> Y5/19(EN_Y)
  [EN_Y] -> Terminator_boundary_DTC8/1
  [N] -> Y6/17(N)
  [shifted_coefficient] -> Y6/18(shifted_coeff)
  [Y15] -> Y6/15(Y15)
  [Y6] -> Y6/6(Y6)
  [Y13] -> Y6/13(Y13)
  [Y5] -> Y6/5(Y5)
  [Y14] -> Y6/14(Y14)
  [Y4] -> Y6/4(Y4)
  [Y7] -> Y6/7(Y7)
  [Y8] -> Y6/8(Y8)
  [Y12] -> Y6/12(Y12)
  [Y2] -> Y6/2(Y2)
  [Y11] -> Y6/11(Y11)
  [Y9] -> Y6/9(Y9)
  [Y3] -> Y6/3(Y3)
  [X] -> Y6/16(X)
  [Y10] -> Y6/10(Y10)
  [Y1] -> Y6/1(Y1)
  Terminator_boundary_DTC8/1 -> Y6/19(EN_Y)
  [EN_Y] -> Terminator_boundary_DTC9/1
  [N] -> Y7/17(N)
  [shifted_coefficient] -> Y7/18(shifted_coeff)
  [Y15] -> Y7/15(Y15)
  [Y6] -> Y7/6(Y6)
  [Y13] -> Y7/13(Y13)
  [Y5] -> Y7/5(Y5)
  [Y14] -> Y7/14(Y14)
  [Y4] -> Y7/4(Y4)
  [Y7] -> Y7/7(Y7)
  [Y8] -> Y7/8(Y8)
  [Y12] -> Y7/12(Y12)
  [Y2] -> Y7/2(Y2)
  [Y11] -> Y7/11(Y11)
  [Y9] -> Y7/9(Y9)
  [Y3] -> Y7/3(Y3)
  [X] -> Y7/16(X)
  [Y10] -> Y7/10(Y10)
  [Y1] -> Y7/1(Y1)
  Terminator_boundary_DTC9/1 -> Y7/19(EN_Y)
  [EN_Y] -> Terminator_boundary_DTC11/1
  [N] -> Y8/17(N)
  [shifted_coefficient] -> Y8/18(shifted_coeff)
  [Y15] -> Y8/15(Y15)
  [Y6] -> Y8/6(Y6)
  [Y13] -> Y8/13(Y13)
  [Y5] -> Y8/5(Y5)
  [Y14] -> Y8/14(Y14)
  [Y4] -> Y8/4(Y4)
  [Y7] -> Y8/7(Y7)
  [Y8] -> Y8/8(Y8)
  [Y12] -> Y8/12(Y12)
  [Y2] -> Y8/2(Y2)
  [Y11] -> Y8/11(Y11)
  [Y9] -> Y8/9(Y9)
  [Y3] -> Y8/3(Y3)
  [X] -> Y8/16(X)
  [Y10] -> Y8/10(Y10)
  [Y1] -> Y8/1(Y1)
  Terminator_boundary_DTC11/1 -> Y8/19(EN_Y)
  [EN_Y] -> Terminator_boundary_DTC12/1
  [N] -> Y9/17(N)
  [shifted_coefficient] -> Y9/18(shifted_coeff)
  [Y15] -> Y9/15(Y15)
  [Y6] -> Y9/6(Y6)
  [Y13] -> Y9/13(Y13)
  [Y5] -> Y9/5(Y5)
  [Y14] -> Y9/14(Y14)
  [Y4] -> Y9/4(Y4)
  [Y7] -> Y9/7(Y7)
  [Y8] -> Y9/8(Y8)
  [Y12] -> Y9/12(Y12)
  [Y2] -> Y9/2(Y2)
  [Y11] -> Y9/11(Y11)
  [Y9] -> Y9/9(Y9)
  [Y3] -> Y9/3(Y3)
  [X] -> Y9/16(X)
  [Y10] -> Y9/10(Y10)
  [Y1] -> Y9/1(Y1)
  Terminator_boundary_DTC12/1 -> Y9/19(EN_Y)
  [EN_Y] -> Terminator_boundary_DTC13/1
  [N] -> Y10/17(N)
  [shifted_coefficient] -> Y10/18(shifted_coeff)
  [Y15] -> Y10/15(Y15)
  [Y6] -> Y10/6(Y6)
  [Y13] -> Y10/13(Y13)
  [Y5] -> Y10/5(Y5)
  [Y14] -> Y10/14(Y14)
  [Y4] -> Y10/4(Y4)
  [Y7] -> Y10/7(Y7)
  [Y8] -> Y10/8(Y8)
  [Y12] -> Y10/12(Y12)
  [Y2] -> Y10/2(Y2)
  [Y11] -> Y10/11(Y11)
  [Y9] -> Y10/9(Y9)
  [Y3] -> Y10/3(Y3)
  [X] -> Y10/16(X)
  [Y10] -> Y10/10(Y10)
  [Y1] -> Y10/1(Y1)
  Terminator_boundary_DTC13/1 -> Y10/19(EN_Y)
  [EN_Y] -> Terminator_boundary_DTC14/1
  [N] -> Y11/17(N)
  [shifted_coefficient] -> Y11/18(shifted_coeff)
  [Y15] -> Y11/15(Y15)
  [Y6] -> Y11/6(Y6)
  [Y13] -> Y11/13(Y13)
  [Y5] -> Y11/5(Y5)
  [Y14] -> Y11/14(Y14)
  [Y4] -> Y11/4(Y4)
  [Y7] -> Y11/7(Y7)
  [Y8] -> Y11/8(Y8)
  [Y12] -> Y11/12(Y12)
  [Y2] -> Y11/2(Y2)
  [Y11] -> Y11/11(Y11)
  [Y9] -> Y11/9(Y9)
  [Y3] -> Y11/3(Y3)
  [X] -> Y11/16(X)
  [Y10] -> Y11/10(Y10)
  [Y1] -> Y11/1(Y1)
  Terminator_boundary_DTC14/1 -> Y11/19(EN_Y)
  [EN_Y] -> Terminator_boundary_DTC15/1
  [N] -> Y12/17(N)
  [shifted_coefficient] -> Y12/18(shifted_coeff)
  [Y15] -> Y12/15(Y15)
  [Y6] -> Y12/6(Y6)
  [Y13] -> Y12/13(Y13)
  [Y5] -> Y12/5(Y5)
  [Y14] -> Y12/14(Y14)
  [Y4] -> Y12/4(Y4)
  [Y7] -> Y12/7(Y7)
  [Y8] -> Y12/8(Y8)
  [Y12] -> Y12/12(Y12)
  [Y2] -> Y12/2(Y2)
  [Y11] -> Y12/11(Y11)
  [Y9] -> Y12/9(Y9)
  [Y3] -> Y12/3(Y3)
  [X] -> Y12/16(X)
  [Y10] -> Y12/10(Y10)
  [Y1] -> Y12/1(Y1)
  Terminator_boundary_DTC15/1 -> Y12/19(EN_Y)
  [EN_Y] -> Terminator_boundary_DTC16/1
  [N] -> Y13/17(N)
  [shifted_coefficient] -> Y13/18(shifted_coeff)
  [Y15] -> Y13/15(Y15)
  [Y6] -> Y13/6(Y6)
  [Y13] -> Y13/13(Y13)
  [Y5] -> Y13/5(Y5)
  [Y14] -> Y13/14(Y14)
  [Y4] -> Y13/4(Y4)
  [Y7] -> Y13/7(Y7)
  [Y8] -> Y13/8(Y8)
  [Y12] -> Y13/12(Y12)
  [Y2] -> Y13/2(Y2)
  [Y11] -> Y13/11(Y11)
  [Y9] -> Y13/9(Y9)
  [Y3] -> Y13/3(Y3)
  [X] -> Y13/16(X)
  [Y10] -> Y13/10(Y10)
  [Y1] -> Y13/1(Y1)
  Terminator_boundary_DTC16/1 -> Y13/19(EN_Y)
  [EN_Y] -> Terminator_boundary_DTC17/1
  [N] -> Y14/17(N)
  [shifted_coefficient] -> Y14/18(shifted_coeff)
  [Y15] -> Y14/15(Y15)
  [Y6] -> Y14/6(Y6)
  [Y13] -> Y14/13(Y13)
  [Y5] -> Y14/5(Y5)
  [Y14] -> Y14/14(Y14)
  [Y4] -> Y14/4(Y4)
  [Y7] -> Y14/7(Y7)
  [Y8] -> Y14/8(Y8)
  [Y12] -> Y14/12(Y12)
  [Y2] -> Y14/2(Y2)
  [Y11] -> Y14/11(Y11)
  [Y9] -> Y14/9(Y9)
  [Y3] -> Y14/3(Y3)
  [X] -> Y14/16(X)
  [Y10] -> Y14/10(Y10)
  [Y1] -> Y14/1(Y1)
  Terminator_boundary_DTC17/1 -> Y14/19(EN_Y)
  [EN_Y] -> Terminator_boundary_DTC18/1
  [N] -> Y15/17(N)
  [shifted_coefficient] -> Y15/18(shifted_coeff)
  [Y15] -> Y15/15(Y15)
  [Y6] -> Y15/6(Y6)
  [Y13] -> Y15/13(Y13)
  [Y5] -> Y15/5(Y5)
  [Y14] -> Y15/14(Y14)
  [Y4] -> Y15/4(Y4)
  [Y7] -> Y15/7(Y7)
  [Y8] -> Y15/8(Y8)
  [Y12] -> Y15/12(Y12)
  [Y2] -> Y15/2(Y2)
  [Y11] -> Y15/11(Y11)
  [Y9] -> Y15/9(Y9)
  [Y3] -> Y15/3(Y3)
  [X] -> Y15/16(X)
  [Y10] -> Y15/10(Y10)
  [Y1] -> Y15/1(Y1)
  Terminator_boundary_DTC18/1 -> Y15/19(EN_Y)
  Terminator_boundary_DTC36/1 -> Switch_2/1
  [EN_X3] -> Switch_1/2
  Switch_1/1 -> [X3]
  Delay2/1 -> Terminator_boundary_DTC35/1
  Delay1/1 -> Terminator_boundary_DTC36/1
  Constant2/1 -> Switch_1/3
  [EN_X4] -> Switch_2/2
  Constant1/1 -> Switch_2/3
  Switch_2/1 -> [X4]
  Pbit_3/1(OUT) -> Delay2/1
  Terminator_boundary_DTC35/1 -> Switch_1/1
  Pbit_4/1(OUT) -> Delay1/1
  Switch_3/1 -> [X5]
  Pbit_5/1(OUT) -> Delay3/1
  Constant3/1 -> Switch_3/3
  [EN_X5] -> Switch_3/2
  Terminator_boundary_DTC37/1 -> Switch_3/1
  Delay3/1 -> Terminator_boundary_DTC37/1
  Pbit_8/1(OUT) -> Delay6/1
  Pbit_9/1(OUT) -> Delay4/1
  Terminator_boundary_DTC38/1 -> Switch_5/1
  Delay6/1 -> Terminator_boundary_DTC38/1
  Switch_5/1 -> [X8]
  Constant9/1 -> Switch_5/3
  [EN_X8] -> Switch_5/2
  Terminator_boundary_DTC39/1 -> Switch_8/1
  Delay4/1 -> Terminator_boundary_DTC39/1
  Switch_9/1 -> [X10]
  [EN_X10] -> Switch_9/2
  Delay7/1 -> Terminator_boundary_DTC41/1
  Constant12/1 -> Switch_9/3
  Constant4/1 -> Switch_8/3
  Terminator_boundary_DTC41/1 -> Switch_9/1
  Terminator_boundary_DTC43/1 -> Switch_7/1
  Switch_8/1 -> [X9]
  [EN_X6] -> Switch_6/2
  Switch_6/1 -> [X6]
  Delay8/1 -> Terminator_boundary_DTC42/1
  Delay5/1 -> Terminator_boundary_DTC43/1
  Constant7/1 -> Switch_6/3
  [EN_X7] -> Switch_7/2
  Constant6/1 -> Switch_7/3
  Switch_7/1 -> [X7]
  Terminator_boundary_DTC42/1 -> Switch_6/1
  Pbit_7/1(OUT) -> Delay5/1
  Pbit_10/1(OUT) -> Delay7/1
  Pbit_6/1(OUT) -> Delay8/1
  [EN_X9] -> Switch_8/2
  Pbit_13/1(OUT) -> Delay11/1
  Pbit_14/1(OUT) -> Delay9/1
  Terminator_boundary_DTC44/1 -> Switch_10/1
  Delay11/1 -> Terminator_boundary_DTC44/1
  Switch_10/1 -> [X13]
  Constant17/1 -> Switch_10/3
  [EN_X13] -> Switch_10/2
  Terminator_boundary_DTC45/1 -> Switch_13/1
  Delay9/1 -> Terminator_boundary_DTC45/1
  Switch_14/1 -> [X15]
  [EN_X15] -> Switch_14/2
  Delay12/1 -> Terminator_boundary_DTC46/1
  Constant18/1 -> Switch_14/3
  Constant13/1 -> Switch_13/3
  Terminator_boundary_DTC46/1 -> Switch_14/1
  Terminator_boundary_DTC48/1 -> Switch_12/1
  Switch_13/1 -> [X14]
  [EN_X11] -> Switch_11/2
  Switch_11/1 -> [X11]
  Delay13/1 -> Terminator_boundary_DTC47/1
  Delay10/1 -> Terminator_boundary_DTC48/1
  Constant15/1 -> Switch_11/3
  [EN_X12] -> Switch_12/2
  Constant14/1 -> Switch_12/3
  Switch_12/1 -> [X12]
  Terminator_boundary_DTC47/1 -> Switch_11/1
  Pbit_12/1(OUT) -> Delay10/1
  Pbit_15/1(OUT) -> Delay12/1
  Pbit_11/1(OUT) -> Delay13/1
  [EN_X14] -> Switch_13/2
  Repeating Sequence Stair/1 -> Math Function1/2
  Product1/1 -> [shifted_coefficient]  "Shifted_coefficient_E0"
  Constant131/1 -> Math Function1/1
  Math Function1/1 -> Product1/2  "Shift_register_output_to_(S)"
  Math Function2/1 -> Product1/1  "E0"
  Constant22/1 -> Math Function2/1
  Constant23/1 -> Math Function2/2

== system Model_without_decision_and_sieve/Enable_Switch ==
  pre_X : Inport  OutDataTypeStr=fixdt(0,1,0)  LockScale=on
  pre_Y : Inport  Port=2  OutDataTypeStr=fixdt(0,1,0)  LockScale=on
  energy : Inport  Port=3  OutDataTypeStr=fixdt(0,1,0)  LockScale=on
  Constant : Constant  Value=0  OutDataTypeStr=fixdt(0,1,0)  LockScale=on
  Switch_1 : Switch  Criteria=u2 ~= 0  OutDataTypeStr=fixdt(0,1,0)  InputSameDT=off
      settings: LockScale=on
  Switch_2 : Switch  Criteria=u2 ~= 0  OutDataTypeStr=fixdt(0,1,0)  InputSameDT=off
      settings: LockScale=on
  EN_X : Outport  OutDataTypeStr=fixdt(0,1,0)  LockScale=on
  EN_Y : Outport  Port=2  OutDataTypeStr=fixdt(0,1,0)  LockScale=on
  wires:
  [energy] -> Switch_1/2
  pre_X/1 -> Switch_1/1
  energy/1 -> [energy]
  Constant/1 -> [zero]
  [zero] -> Switch_1/3
  pre_Y/1 -> Switch_2/1
  [zero] -> Switch_2/3
  [energy] -> Switch_2/2
  Switch_1/1 -> EN_X/1
  Switch_2/1 -> EN_Y/1

== system Model_without_decision_and_sieve/Pbit_1 ==
  note: without a delay block, this block naturally gets the output of EN=1 block's output @ EN=0 so an unit delay is naturally applied
  note: random value does not change when EN=0
  note: so EN=0 block simply passes the same OUT value to a multiport switch
  IN : Inport
  EN : Inport  Port=2
  Cast To Double : DataTypeConversion  OutDataTypeStr=double  SaturateOnIntegerOverflow=off  RndMeth=Floor
  Cast To Double1 : DataTypeConversion  OutDataTypeStr=double  SaturateOnIntegerOverflow=off  RndMeth=Floor
  EN=0 Block : Subsystem  TreatAsAtomicUnit=on
  EN=1 Block : Subsystem  TreatAsAtomicUnit=on
  If : If
  Multiport Switch : MultiPortSwitch  DataPortOrder=Zero-based contiguous  Inputs=2  zeroidx=on  SaturateOnIntegerOverflow=off  InputSameDT=off
  OUT : Outport
  wires:
  Cast To Double1/1 -> Multiport Switch/2
  Cast To Double/1 -> Multiport Switch/3
  [EN] -> Multiport Switch/1
  EN=0 Block/1(Out1) -> Cast To Double1/1  "OUT_EN=0"
  EN=1 Block/1(OUT) -> EN=0 Block/1(IN), Cast To Double/1  "OUT_EN=1"
  If/2 -> EN=0 Block/Action
  If/1 -> EN=1 Block/Action
  Multiport Switch/1 -> OUT/1  "OUT_MUX"
  EN/1 -> If/1, [EN]
  IN/1 -> EN=1 Block/1(IN)

== system Model_without_decision_and_sieve/Pbit_10 ==
  note: without a delay block, this block naturally gets the output of EN=1 block's output @ EN=0 so an unit delay is naturally applied
  note: random value does not change when EN=0
  note: so EN=0 block simply passes the same OUT value to a multiport switch
  IN : Inport
  EN : Inport  Port=2
  Cast To Double : DataTypeConversion  OutDataTypeStr=double  SaturateOnIntegerOverflow=off  RndMeth=Floor
  Cast To Double1 : DataTypeConversion  OutDataTypeStr=double  SaturateOnIntegerOverflow=off  RndMeth=Floor
  EN=0 Block : Subsystem  TreatAsAtomicUnit=on
  EN=1 Block : Subsystem  TreatAsAtomicUnit=on
  If : If
  Multiport Switch : MultiPortSwitch  DataPortOrder=Zero-based contiguous  Inputs=2  zeroidx=on  SaturateOnIntegerOverflow=off  InputSameDT=off
  OUT : Outport
  wires:
  Cast To Double1/1 -> Multiport Switch/2
  Cast To Double/1 -> Multiport Switch/3
  [EN] -> Multiport Switch/1
  EN=0 Block/1(Out1) -> Cast To Double1/1  "OUT_EN=0"
  EN=1 Block/1(OUT) -> EN=0 Block/1(IN), Cast To Double/1  "OUT_EN=1"
  If/2 -> EN=0 Block/Action
  If/1 -> EN=1 Block/Action
  Multiport Switch/1 -> OUT/1  "OUT_MUX"
  EN/1 -> If/1, [EN]
  IN/1 -> EN=1 Block/1(IN)

== system Model_without_decision_and_sieve/Pbit_11 ==
  note: without a delay block, this block naturally gets the output of EN=1 block's output @ EN=0 so an unit delay is naturally applied
  note: random value does not change when EN=0
  note: so EN=0 block simply passes the same OUT value to a multiport switch
  IN : Inport
  EN : Inport  Port=2
  Cast To Double : DataTypeConversion  OutDataTypeStr=double  SaturateOnIntegerOverflow=off  RndMeth=Floor
  Cast To Double1 : DataTypeConversion  OutDataTypeStr=double  SaturateOnIntegerOverflow=off  RndMeth=Floor
  EN=0 Block : Subsystem  TreatAsAtomicUnit=on
  EN=1 Block : Subsystem  TreatAsAtomicUnit=on
  If : If
  Multiport Switch : MultiPortSwitch  DataPortOrder=Zero-based contiguous  Inputs=2  zeroidx=on  SaturateOnIntegerOverflow=off  InputSameDT=off
  OUT : Outport
  wires:
  Cast To Double1/1 -> Multiport Switch/2
  Cast To Double/1 -> Multiport Switch/3
  [EN] -> Multiport Switch/1
  EN=0 Block/1(Out1) -> Cast To Double1/1  "OUT_EN=0"
  EN=1 Block/1(OUT) -> EN=0 Block/1(IN), Cast To Double/1  "OUT_EN=1"
  If/2 -> EN=0 Block/Action
  If/1 -> EN=1 Block/Action
  Multiport Switch/1 -> OUT/1  "OUT_MUX"
  EN/1 -> If/1, [EN]
  IN/1 -> EN=1 Block/1(IN)

== system Model_without_decision_and_sieve/Pbit_12 ==
  note: without a delay block, this block naturally gets the output of EN=1 block's output @ EN=0 so an unit delay is naturally applied
  note: random value does not change when EN=0
  note: so EN=0 block simply passes the same OUT value to a multiport switch
  IN : Inport
  EN : Inport  Port=2
  Cast To Double : DataTypeConversion  OutDataTypeStr=double  SaturateOnIntegerOverflow=off  RndMeth=Floor
  Cast To Double1 : DataTypeConversion  OutDataTypeStr=double  SaturateOnIntegerOverflow=off  RndMeth=Floor
  EN=0 Block : Subsystem  TreatAsAtomicUnit=on
  EN=1 Block : Subsystem  TreatAsAtomicUnit=on
  If : If
  Multiport Switch : MultiPortSwitch  DataPortOrder=Zero-based contiguous  Inputs=2  zeroidx=on  SaturateOnIntegerOverflow=off  InputSameDT=off
  OUT : Outport
  wires:
  Cast To Double1/1 -> Multiport Switch/2
  Cast To Double/1 -> Multiport Switch/3
  [EN] -> Multiport Switch/1
  EN=0 Block/1(Out1) -> Cast To Double1/1  "OUT_EN=0"
  EN=1 Block/1(OUT) -> EN=0 Block/1(IN), Cast To Double/1  "OUT_EN=1"
  If/2 -> EN=0 Block/Action
  If/1 -> EN=1 Block/Action
  Multiport Switch/1 -> OUT/1  "OUT_MUX"
  EN/1 -> If/1, [EN]
  IN/1 -> EN=1 Block/1(IN)

== system Model_without_decision_and_sieve/Pbit_13 ==
  note: so EN=0 block simply passes the same OUT value to a multiport switch
  note: random value does not change when EN=0
  note: without a delay block, this block naturally gets the output of EN=1 block's output @ EN=0 so an unit delay is naturally applied
  IN : Inport
  EN : Inport  Port=2
  Cast To Double : DataTypeConversion  OutDataTypeStr=double  SaturateOnIntegerOverflow=off  RndMeth=Floor
  Cast To Double1 : DataTypeConversion  OutDataTypeStr=double  SaturateOnIntegerOverflow=off  RndMeth=Floor
  EN=0 Block : Subsystem  TreatAsAtomicUnit=on
  EN=1 Block : Subsystem  TreatAsAtomicUnit=on
  If : If
  Multiport Switch : MultiPortSwitch  DataPortOrder=Zero-based contiguous  Inputs=2  zeroidx=on  SaturateOnIntegerOverflow=off  InputSameDT=off
  OUT : Outport
  wires:
  IN/1 -> EN=1 Block/1(IN)
  EN/1 -> [EN], If/1
  Multiport Switch/1 -> OUT/1  "OUT_MUX"
  If/1 -> EN=1 Block/Action
  If/2 -> EN=0 Block/Action
  EN=1 Block/1(OUT) -> Cast To Double/1, EN=0 Block/1(IN)  "OUT_EN=1"
  EN=0 Block/1(Out1) -> Cast To Double1/1  "OUT_EN=0"
  [EN] -> Multiport Switch/1
  Cast To Double/1 -> Multiport Switch/3
  Cast To Double1/1 -> Multiport Switch/2

== system Model_without_decision_and_sieve/Pbit_14 ==
  note: so EN=0 block simply passes the same OUT value to a multiport switch
  note: random value does not change when EN=0
  note: without a delay block, this block naturally gets the output of EN=1 block's output @ EN=0 so an unit delay is naturally applied
  IN : Inport
  EN : Inport  Port=2
  Cast To Double : DataTypeConversion  OutDataTypeStr=double  SaturateOnIntegerOverflow=off  RndMeth=Floor
  Cast To Double1 : DataTypeConversion  OutDataTypeStr=double  SaturateOnIntegerOverflow=off  RndMeth=Floor
  EN=0 Block : Subsystem  TreatAsAtomicUnit=on
  EN=1 Block : Subsystem  TreatAsAtomicUnit=on
  If : If
  Multiport Switch : MultiPortSwitch  DataPortOrder=Zero-based contiguous  Inputs=2  zeroidx=on  SaturateOnIntegerOverflow=off  InputSameDT=off
  OUT : Outport
  wires:
  IN/1 -> EN=1 Block/1(IN)
  EN/1 -> [EN], If/1
  Multiport Switch/1 -> OUT/1  "OUT_MUX"
  If/1 -> EN=1 Block/Action
  If/2 -> EN=0 Block/Action
  EN=1 Block/1(OUT) -> Cast To Double/1, EN=0 Block/1(IN)  "OUT_EN=1"
  EN=0 Block/1(Out1) -> Cast To Double1/1  "OUT_EN=0"
  [EN] -> Multiport Switch/1
  Cast To Double/1 -> Multiport Switch/3
  Cast To Double1/1 -> Multiport Switch/2

== system Model_without_decision_and_sieve/Pbit_15 ==
  note: without a delay block, this block naturally gets the output of EN=1 block's output @ EN=0 so an unit delay is naturally applied
  note: random value does not change when EN=0
  note: so EN=0 block simply passes the same OUT value to a multiport switch
  IN : Inport
  EN : Inport  Port=2
  Cast To Double : DataTypeConversion  OutDataTypeStr=double  SaturateOnIntegerOverflow=off  RndMeth=Floor
  Cast To Double1 : DataTypeConversion  OutDataTypeStr=double  SaturateOnIntegerOverflow=off  RndMeth=Floor
  EN=0 Block : Subsystem  TreatAsAtomicUnit=on
  EN=1 Block : Subsystem  TreatAsAtomicUnit=on
  If : If
  Multiport Switch : MultiPortSwitch  DataPortOrder=Zero-based contiguous  Inputs=2  zeroidx=on  SaturateOnIntegerOverflow=off  InputSameDT=off
  OUT : Outport
  wires:
  Cast To Double1/1 -> Multiport Switch/2
  Cast To Double/1 -> Multiport Switch/3
  [EN] -> Multiport Switch/1
  EN=0 Block/1(Out1) -> Cast To Double1/1  "OUT_EN=0"
  EN=1 Block/1(OUT) -> EN=0 Block/1(IN), Cast To Double/1  "OUT_EN=1"
  If/2 -> EN=0 Block/Action
  If/1 -> EN=1 Block/Action
  Multiport Switch/1 -> OUT/1  "OUT_MUX"
  EN/1 -> If/1, [EN]
  IN/1 -> EN=1 Block/1(IN)
